simulink model "Cartesian_first"  (R2021a)
settings: Solver=VariableStepAuto  StartTime=0.0  StopTime=20  RelTol=1e-3
libraries: robotmaniplib x4, robotcorelib x2
settings Model: Creator=ASUS  LastModifiedBy=ASUS

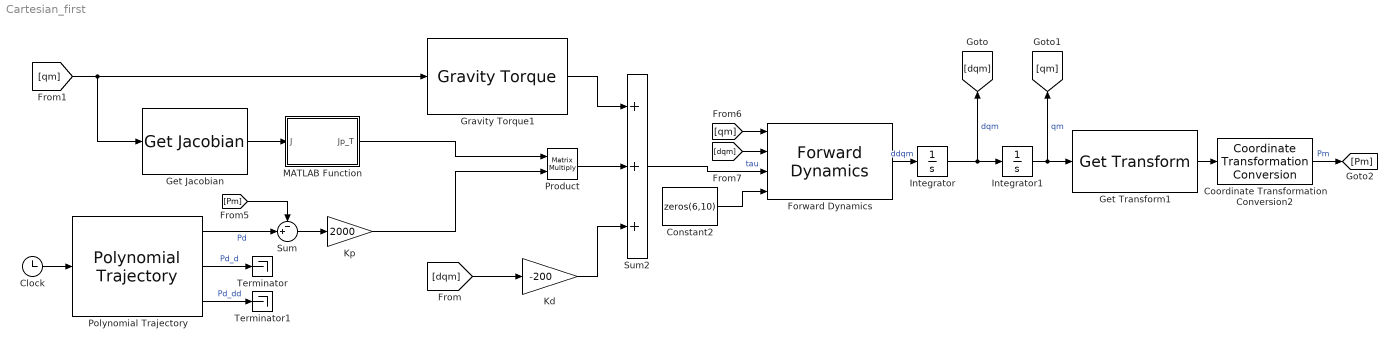
== system Cartesian_first ==
  Clock : Clock
  Constant2 : Constant  Value=zeros(6,10)
  Coordinate Transformation Conversion2 : robotcorelib/Coordinate Transformation Conversion  InputRepresentation=Homogeneous Transformation  InputEulerSequence=ZYX  ShowTrVecInputPort=on  OutputRepresentation=Translation Vector  OutputEulerSequence=ZYX  ShowTrVecOutputPort=on  SimulateUsing=Code generation
      settings: SourceProductBaseCode=NV,RO,RR,UV
  Forward Dynamics : robotmaniplib/Forward Dynamics  RigidBodyTree=robot  SimulateUsing=Code generation
  Get Jacobian : robotmaniplib/Get Jacobian  RigidBodyTree=robot  EndEffector=tool0  SimulateUsing=Code generation
      settings: SourceProductBaseCode=RO
  Get Transform1 : robotmaniplib/Get Transform  RigidBodyTree=robot  SourceBody=tool0  TargetBody=world  SimulateUsing=Code generation
  Gravity Torque1 : robotmaniplib/Gravity Torque  RigidBodyTree=robot  SimulateUsing=Code generation
  Integrator : Integrator
  Integrator1 : Integrator
  Kd : Gain  Gain=-200
  Kp : Gain  Gain=2000
  MATLAB Function : MATLAB Function  TreatAsAtomicUnit=on
  Polynomial Trajectory : robotcorelib/Polynomial Trajectory  WaypointSource=Internal  Waypoints=[ 0.1 0.1; 0.2 0.2; 0.3 0.3]  TimePoints=[ 0, 0.01 ]  TimeInterval=[ 1, 4 ]  Method=Cubic Polynomial  ParameterSource=Internal  VelocityBoundaryCondition=zeros( 3, 2 )  AccelerationBoundaryCondition=zeros( 2, 5 )  SimulateUsing=Interpreted execution
  Product : Product  Multiplication=Matrix(*)
  Sum : Sum  Inputs=-+|
  Sum2 : Sum  Inputs=+++
  Terminator : Terminator
  Terminator1 : Terminator
  wires:
  [dqm] -> Kd/1
  Kd/1 -> Sum2/3
  Get Jacobian/1 -> MATLAB Function/1(J)
  [qm] -> Get Jacobian/1, Gravity Torque1/1
  Kp/1 -> Product/2
  Product/1 -> Sum2/2
  Polynomial Trajectory/2 -> Terminator/1  "Pd_d"
  Get Transform1/1 -> Coordinate Transformation Conversion2/1
  Coordinate Transformation Conversion2/1 -> [Pm]  "Pm"
  MATLAB Function/1(Jp_T) -> Product/1
  Polynomial Trajectory/1 -> Sum/2  "Pd"
  Gravity Torque1/1 -> Sum2/1
  Clock/1 -> Polynomial Trajectory/1
  Integrator/1 -> [dqm], Integrator1/1  "dqm"
  Integrator1/1 -> Get Transform1/1, [qm]  "qm"
  Constant2/1 -> Forward Dynamics/4
  [qm] -> Forward Dynamics/1
  Sum/1 -> Kp/1
  [Pm] -> Sum/1
  Polynomial Trajectory/3 -> Terminator1/1  "Pd_dd"
  Sum2/1 -> Forward Dynamics/3  "tau"
  [dqm] -> Forward Dynamics/2
  Forward Dynamics/1 -> Integrator/1  "ddqm"

== matlab function Cartesian_first/MATLAB Function ==
  data: J input; Jp_T output
function Jp_T = fcn(J)

Jp_T = J(4:6,:)';

end
